simulink model "full"  (R2021b)
settings: Solver=VariableStepAuto  StartTime=0.0  StopTime=10.0  RelTol=1e-3
settings Model: Creator=anton  LastModifiedBy=anton

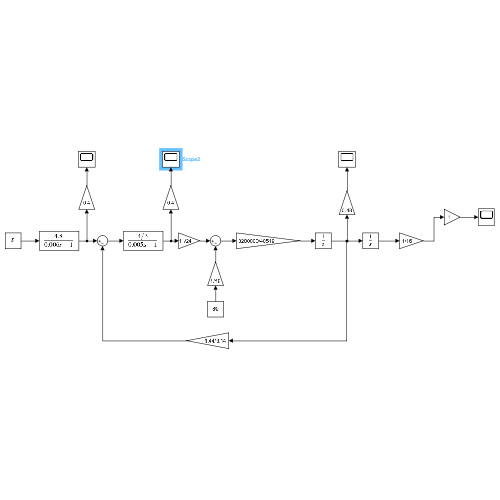
[thumbnail: Simulink's stored preview of the top-level diagram]
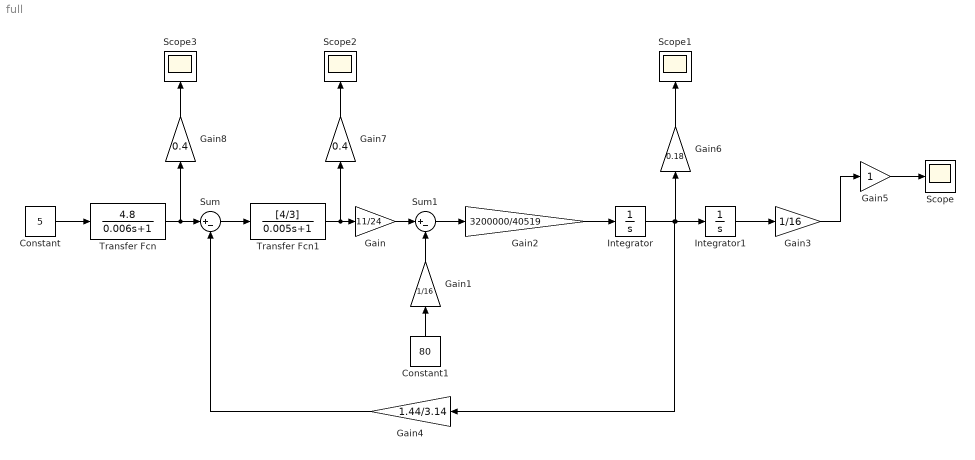
== system full ==
  Constant : Constant  Value=5
  Constant1 : Constant  Value=80
  Gain : Gain  Gain=11/24
  Gain1 : Gain  Gain=1/16
  Gain2 : Gain  Gain=3200000/40519
  Gain3 : Gain  Gain=1/16
  Gain4 : Gain  Gain=1.44/3.14
  Gain5 : Gain
  Gain6 : Gain  Gain=0.18
  Gain7 : Gain  Gain=0.4
  Gain8 : Gain  Gain=0.4
  Integrator : Integrator
  Integrator1 : Integrator
  Scope{,1..3} (4 alike) : Scope
  Sum : Sum  Inputs=|+-
  Sum1 : Sum  Inputs=|+-
  Transfer Fcn : TransferFcn  Numerator=[4.8]  Denominator=[0.006 1]
  Transfer Fcn1 : TransferFcn  Numerator=[4/3]  Denominator=[0.005 1]
  wires:
  Constant/1 -> Transfer Fcn/1
  Transfer Fcn/1 -> Gain8/1, Sum/1
  Sum/1 -> Transfer Fcn1/1
  Transfer Fcn1/1 -> Gain7/1, Gain/1
  Gain/1 -> Sum1/1
  Constant1/1 -> Gain1/1
  Gain1/1 -> Sum1/2
  Sum1/1 -> Gain2/1
  Gain2/1 -> Integrator/1
  Integrator/1 -> Gain6/1, Integrator1/1, Gain4/1
  Integrator1/1 -> Gain3/1
  Gain4/1 -> Sum/2
  Gain3/1 -> Gain5/1
  Gain5/1 -> Scope/1
  Gain6/1 -> Scope1/1
  Gain7/1 -> Scope2/1
  Gain8/1 -> Scope3/1
